simulink model "HDLHeaderRemoveRepetition"  (R2024a)
settings: Solver=VariableStepAuto  StartTime=0.0  StopTime=stopTime  RelTol=1e-3
undefined symbols (not defined in the file): CONST
libraries: dspsrcs4 x2, whdlutilities x1, HDL_ieee_8021513 x1
settings Model: Creator=cotti  LastModifiedBy=cotti

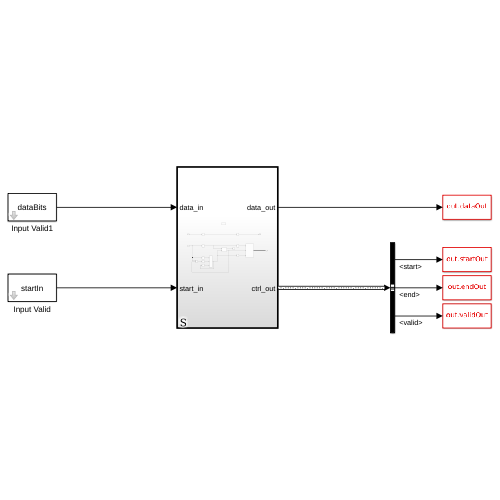
[thumbnail: Simulink's stored preview of the top-level diagram]
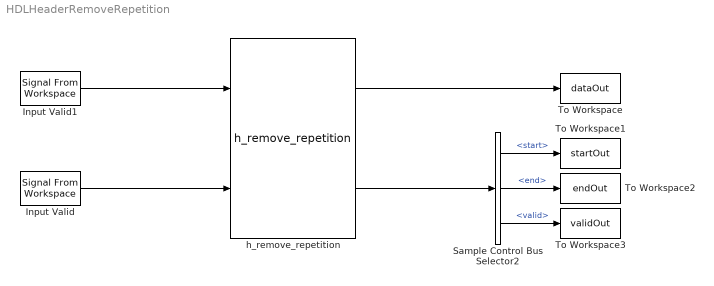
== system HDLHeaderRemoveRepetition ==
  Input Valid : dspsrcs4/Signal From Workspace  X=startIn  Ts=1/CONST.fs  nsamps=1  OutputAfterFinalValue=Setting to zero  ignoreOrWarnInputAndFrameLengths=off  OutputFrames=off
  Input Valid1 : dspsrcs4/Signal From Workspace  X=dataBits  Ts=1/CONST.fs  nsamps=1  OutputAfterFinalValue=Setting to zero  ignoreOrWarnInputAndFrameLengths=off  OutputFrames=off
  Sample Control Bus Selector2 : whdlutilities/Sample Control Bus Selector  OutputSignals=start,end,valid
  To Workspace : ToWorkspace  VariableName=dataOut  SampleTime=1/CONST.fs
      settings: Save2DSignal=2-D array (concatenate along first dimension)
  To Workspace1 : ToWorkspace  VariableName=startOut  SampleTime=1/CONST.fs
      settings: Save2DSignal=2-D array (concatenate along first dimension)
  To Workspace2 : ToWorkspace  VariableName=endOut  SampleTime=1/CONST.fs
      settings: Save2DSignal=2-D array (concatenate along first dimension)
  To Workspace3 : ToWorkspace  VariableName=validOut  SampleTime=1/CONST.fs
      settings: Save2DSignal=2-D array (concatenate along first dimension)
  h_remove_repetition : HDL_ieee_8021513/h_remove_repetition  SystemSampleTime=-1  VariantActivationTime=update diagram  AllowFlexibleInterface=on  Latency=0  AutoFrameSizeCalculation=off
      settings: SourceProductName=HDL IEEE 8021513
  wires:
  Input Valid/1 -> h_remove_repetition/2
  Input Valid1/1 -> h_remove_repetition/1
  h_remove_repetition/2 -> Sample Control Bus Selector2/1
  Sample Control Bus Selector2/3 -> To Workspace3/1  "<valid>"
  h_remove_repetition/1 -> To Workspace/1
  Sample Control Bus Selector2/2 -> To Workspace2/1  "<end>"
  Sample Control Bus Selector2/1 -> To Workspace1/1  "<start>"
